simulink model "last circuit"  (R2016a)
settings: Solver=VariableStepAuto  StartTime=0.0  StopTime=20  RelTol=1e-3
libraries: powerlib x15, powerlib_meascontrol x1
settings Model: Creator=abdurrahman  LastModifiedBy=abdurrahman

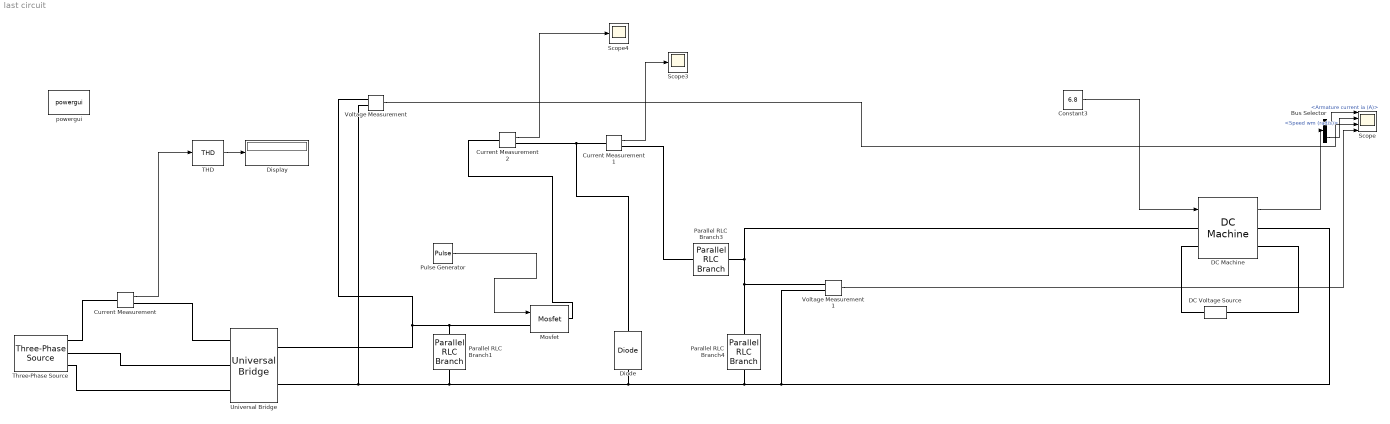
== system last circuit ==
  Bus Selector : BusSelector  OutputSignals=Armature current ia (A),Speed wm (rad/s)
  Constant3 : Constant  Value=6.8
  Current Measurement : powerlib/Measurements/Current Measurement  PhasorSimulation=off  OutputType=Complex  PSBequivalent=0
  Current Measurement1 : powerlib/Measurements/Current Measurement  PhasorSimulation=off  OutputType=Complex  PSBequivalent=0
  Current Measurement2 : powerlib/Measurements/Current Measurement  PhasorSimulation=off  OutputType=Complex  PSBequivalent=0
  DC Machine : powerlib/Machines/DC Machine  PresetModel=No  MechanicalLoad=Torque TL  FieldType=Wound  ShowDetailedParameters=on  MeasurementBus=off  RLa="[ 28  0.0133]"  RLf="[ 8460  6.4]"  Laf=2  MachineConstant=Torque constant (N.m/A)  Ke=1.8  Kt=1.8  J=0.01  Bm=0  Tf=0  w0=1  Ifinit=1  TsPowergui=0  TsBlock=-1
  DC Voltage Source : powerlib/Electrical Sources/DC Voltage Source  Amplitude=220  Measurements=None
  Diode : powerlib/Power Electronics/Diode  Ron=0.001  Lon=0  Vf=0.8  IC=0  UseSnubber=off  Rs=500  Cs=250e-9  Measurements=off
  Display : Display
  Mosfet : powerlib/Power Electronics/Mosfet  Ron=0.1  Lon=0  Rd=0.01  Vfd=0  IC=0  Rs=1e5  Cs=inf  Measurements=off
  Parallel RLC Branch1 : powerlib/Elements/Parallel RLC Branch  LConnTagsString=a  RConnTagsString=__new0  BranchType=C  Resistance=1  Inductance=1e-3  SetiL0=off  InitialCurrent=0  Capacitance=400e-6  Setx0=off  InitialVoltage=0  Measurements=None
  Parallel RLC Branch3 : powerlib/Elements/Parallel RLC Branch  LConnTagsString=a  RConnTagsString=__new0  BranchType=L  Resistance=1  Inductance=0.023  SetiL0=off  InitialCurrent=0  Capacitance=100e-6  Setx0=off  InitialVoltage=0  Measurements=None
  Parallel RLC Branch4 : powerlib/Elements/Parallel RLC Branch  LConnTagsString=a  RConnTagsString=__new0  BranchType=C  Resistance=1  Inductance=1e-3  SetiL0=off  InitialCurrent=0  Capacitance=680e-6  Setx0=off  InitialVoltage=0  Measurements=None
  Pulse Generator : DiscretePulseGenerator  PulseType=Time based  Amplitude=5  Period=1/30000  PulseWidth=10
  Scope : Scope  NumInputPorts=4
  Scope3 : Scope
  Scope4 : Scope
  THD : powerlib_meascontrol/Measurements/THD  Freq=50  Ts=0
  Three-Phase Source : powerlib/Electrical Sources/Three-Phase Source  InternalConnection=Yg  VoltagePhases=off  Voltage=400  PhaseAngle=0  Voltage_phases=[25e3 25e3 25e3]/sqrt(3)  PhaseAngles_phases=[0 -120 +120]  Frequency=50  NonIdealSource=on  SpecifyImpedance=off  Resistance=0.1  Inductance=0.0001  ShortCircuitLevel=100e6  BaseVoltage=25e3  XRratio=7  BusType=swing  Pref=10e3  Qref=0  Prefabc=[10e3, 10e3, 10e3]  Qrefabc=[0, 0, 0]  Qmin=-inf  Qmax=inf
  Universal Bridge : powerlib/Power Electronics/Universal Bridge  Arms=3  SnubberResistance=1e5  SnubberCapacitance=inf  Device=Diodes  Ron=20e-3  Lon=0  ForwardVoltages="[  0  0  ]"  ForwardVoltage=0.8  GTOparameters=[ 10e-6 , 20e-6 ]  IGBTparameters=[ 1e-6 , 2e-6 ]  Measurements=None  Measurements_2=None  converterType=Rectifier
  Voltage Measurement : powerlib/Measurements/Voltage Measurement  PhasorSimulation=off  OutputType=Complex  PSBequivalent=0
  Voltage Measurement1 : powerlib/Measurements/Voltage Measurement  PhasorSimulation=off  OutputType=Complex  PSBequivalent=0
  powergui : powerlib/powergui  Priority=1  SimulationMode=Continuous  SolverType=Tustin/Backward Euler (TBE)  SampleTime=50e-6  frequency=60  SPID=on  DisableSnubberDevices=on  DisableRonSwitches=on  DisableVfSwitches=on  SwTol=0  DisplayEquations=on  Interpol=off  ExternalGateDelay=off  methode=off  Ts=10  FunctionMessages=off  echomessages=off  HookPort=off  EnableUseOfTLC=off  x0status=blocks  frequencyindice=0  Pbase=100e6  ErrMax=1e-4  Iterations=50  UnitsV=kV  UnitsW=MW  buscounter=0  RestoreLinks=warning  ResistiveCurrentMeasurement=off  Frange=[0:2:500]  Ylog=off  Xlog=on  ShowGrid=off  save=off  variable=ZData  structure=0  ZoomFFT=off  StartTime=0.0  cycles=1  DisplayStyle=1  fundamental=60  FreqAxis=off  MaxFrequency=1000  frequencyindicesteady=1  RmsSteady=1  display=off
  wires:
  Current Measurement/1 -> THD/1
  Pulse Generator/1 -> Mosfet/1
  Current Measurement1/1 -> Scope3/1
  Current Measurement2/1 -> Scope4/1
  Constant3/1 -> DC Machine/1
  DC Machine/1 -> Bus Selector/1
  THD/1 -> Display/1
  Voltage Measurement1/1 -> Scope/4
  Voltage Measurement/1 -> Scope/3
  Bus Selector/1 -> Scope/1  "<Armature current ia (A)>"
  Bus Selector/2 -> Scope/2  "<Speed wm (rad/s)>"
  connections:
  Universal Bridge/LConn3 -- Three-Phase Source/RConn3
  Three-Phase Source/RConn2 -- Universal Bridge/LConn2
  Voltage Measurement/LConn1 -- Universal Bridge/RConn1 -- Mosfet/LConn1 -- Parallel RLC Branch1/LConn1
  Universal Bridge/RConn2 -- Voltage Measurement/LConn2 -- DC Machine/RConn1 -- Voltage Measurement1/LConn2 -- Parallel RLC Branch4/RConn1 -- Diode/LConn1 -- Parallel RLC Branch1/RConn1
  Three-Phase Source/RConn1 -- Current Measurement/LConn1
  Current Measurement/RConn1 -- Universal Bridge/LConn1
  Parallel RLC Branch3/LConn1 -- DC Machine/LConn1 -- Parallel RLC Branch4/LConn1 -- Voltage Measurement1/LConn1
  Current Measurement2/RConn1 -- Diode/RConn1 -- Current Measurement1/LConn1
  Current Measurement1/RConn1 -- Parallel RLC Branch3/RConn1
  Current Measurement2/LConn1 -- Mosfet/RConn1
  DC Voltage Source/RConn1 -- DC Machine/LConn2
  DC Voltage Source/LConn1 -- DC Machine/RConn2
